simulink model "normal_"  (R2018a)
settings: Solver=VariableStepAuto  StartTime=0.0  StopTime=5  RelTol=1e-3
settings Model: Creator=80741  LastModifiedBy=80741

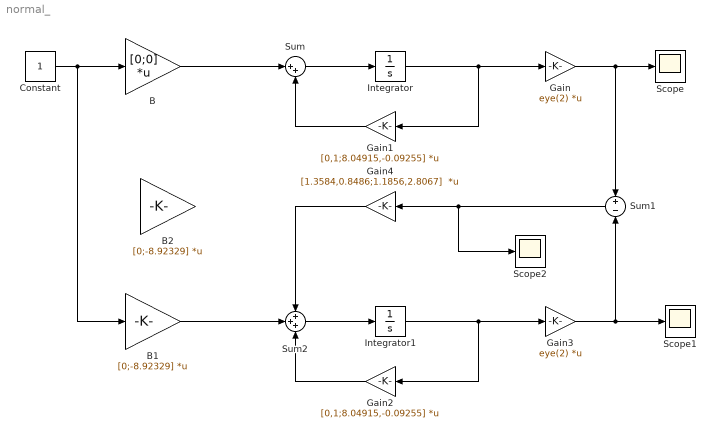
== system normal_ ==
  B : Gain  Gain=[0;0]  Multiplication=Matrix(K*u) (u vector)
  B1 : Gain  Gain=[0;-8.92329]  Multiplication=Matrix(K*u) (u vector)
  B2 : Gain  Gain=[0;-8.92329]  Multiplication=Matrix(K*u) (u vector)
  Constant : Constant
  Gain : Gain  Gain=eye(2)  Multiplication=Matrix(K*u) (u vector)
  Gain1 : Gain  Gain=[0,1;8.04915,-0.09255]  Multiplication=Matrix(K*u) (u vector)
  Gain2 : Gain  Gain=[0,1;8.04915,-0.09255]  Multiplication=Matrix(K*u) (u vector)
  Gain3 : Gain  Gain=eye(2)  Multiplication=Matrix(K*u) (u vector)
  Gain4 : Gain  Gain=[1.3584,0.8486;1.1856,2.8067]  Multiplication=Matrix(K*u) (u vector)
  Integrator : Integrator
  Integrator1 : Integrator
  Scope : Scope
  Scope1 : Scope
  Scope2 : Scope
  Sum : Sum  Inputs=|++
  Sum1 : Sum  Inputs=+-
  Sum2 : Sum  Inputs=+++
  wires:
  B/1 -> Sum/1
  Sum/1 -> Integrator/1
  Integrator/1 -> Gain1/1, Gain/1
  Gain/1 -> Sum1/1, Scope/1
  Gain1/1 -> Sum/2
  Constant/1 -> B/1, B1/1
  Integrator1/1 -> Gain3/1, Gain2/1
  Gain3/1 -> Scope1/1, Sum1/2
  Sum1/1 -> Scope2/1, Gain4/1
  Gain4/1 -> Sum2/1
  Gain2/1 -> Sum2/3
  B1/1 -> Sum2/2
  Sum2/1 -> Integrator1/1
